simulink subsystem "RLC_Series"  (R2022b)
settings: Solver=VariableStepAuto  StartTime=0.0  StopTime=10.0  RelTol=1e-3
model mask{R=10, L=0.01, C=100e-6}
  mask prompts: R "Resistance (Ohm)"; L "inductive (H)"; C "Capacitance (F)"
settings Model: Creator=MAAM  LastModifiedBy=MAAM

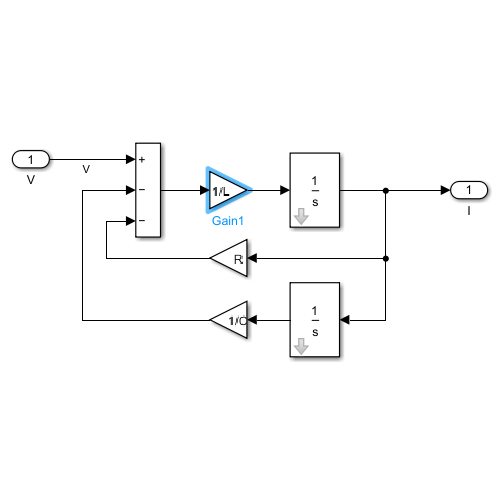
[thumbnail: Simulink's stored preview of the top-level diagram]
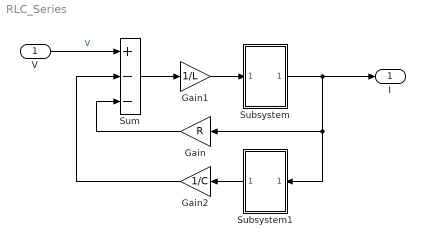
== system RLC_Series ==
  V : Inport
  Gain : Gain  Gain=R
  Gain1 : Gain  Gain=1/L
  Gain2 : Gain  Gain=1/C
  Subsystem : Subsystem  ReferencedSubsystem=Integrator  Gain=1.0  Init=0  SampleTime=1e-6  Ts=auto
  Subsystem1 : Subsystem  ReferencedSubsystem=Integrator  Gain=1.0  Init=0  SampleTime=1e-6  Ts=auto
  Sum : Sum  Inputs=+--
  I : Outport
  wires:
  V/1 -> Sum/1  "V"
  Sum/1 -> Gain1/1
  Gain/1 -> Sum/3
  Gain2/1 -> Sum/2
  Subsystem1/1 -> Gain2/1
  Subsystem/1 -> I/1, Gain/1, Subsystem1/1
  Gain1/1 -> Subsystem/1
